simulink model "test_firs"  (Simulink 6.2)
settings: Solver=ode45  StartTime=0.0  StopTime=500  RelTol=1e-3
undefined symbols (not defined in the file or in its folder): now, pfb_coefs
libraries: xbsIndex_r3 x151, pfb_library x1, simulink x1
(part 3 of 3)

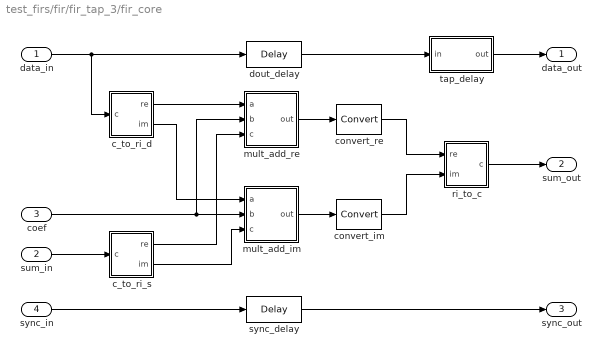
== system test_firs/fir/fir_tap_3/fir_core ==
  data_in : Inport  Port=1  LatchInput=off
  sum_in : Inport  Port=2  LatchInput=off
  coef : Inport  Port=3  LatchInput=off
  sync_in : Inport  Port=4  LatchInput=off
  c_to_ri_d : Subsystem  mask(Complex to Real-Imag){n_bits=8, bin_pt=7}
      mask prompts: n_bits "Bit Width"; bin_pt "Binary Point"
      mask help: Outputs real and imaginary components of a complex input.
      settings: AttributesFormatString=8_7 r/i
      mask Help:
      | <pre>
      | Description::
      | 
      | Outputs real and imaginary components of a complex input.
      | Useful for simplifying interconnects.
      | See also: Real-Imag to Complex (ri_to_c)
      | 
      | Mask Parameters::
      | 
      | Bit Width (n_bits): Specifies the width of the real/imaginary components.
      | Assumed equal for both components.
      | 
      | Binary Point (bin_pt): Specifies the binary point location in the real/imaginary components.
      | Assumed equal for both components.
      | </pre>
  c_to_ri_s : Subsystem  mask(Complex to Real-Imag){n_bits=17, bin_pt=15}
      mask prompts: n_bits "Bit Width"; bin_pt "Binary Point"
      mask help: Outputs real and imaginary components of a complex input.
      settings: AttributesFormatString=17_15 r/i
      mask Help:
      | <pre>
      | Description::
      | 
      | Outputs real and imaginary components of a complex input.
      | Useful for simplifying interconnects.
      | See also: Real-Imag to Complex (ri_to_c)
      | 
      | Mask Parameters::
      | 
      | Bit Width (n_bits): Specifies the width of the real/imaginary components.
      | Assumed equal for both components.
      | 
      | Binary Point (bin_pt): Specifies the binary point location in the real/imaginary components.
      | Assumed equal for both components.
      | </pre>
  convert_im : xbsIndex_r3/Convert  arith_type="Signed  (2's comp)"  n_bits=17  bin_pt=15  quantization=Truncate  overflow=Wrap  latency=0  explicit_period=off  period=1  dbl_ovrd=off  show_param=on  inserted_by_tool=off  pipeline=on
      settings: xl_area=[0, 0, 0, 0, 0, 0, 0]
  convert_re : xbsIndex_r3/Convert  arith_type="Signed  (2's comp)"  n_bits=17  bin_pt=15  quantization=Truncate  overflow=Wrap  latency=0  explicit_period=off  period=1  dbl_ovrd=off  show_param=on  inserted_by_tool=off  pipeline=on
      settings: xl_area=[0, 0, 0, 0, 0, 0, 0]
  dout_delay : xbsIndex_r3/Delay  latency=4  reg_retiming=off  explicit_period=off  period=1  en=off  accept_only_valid=off  init_zero=on  dbl_ovrd=off  show_param=off
      settings: xl_area=[0, 0, 0, 0, 0, 0, 0]
  mult_add_im : Subsystem  mask(Multiply Add Block){mult_latency=3, add_latency=1, add_bypass=off}
      mask prompts: mult_latency "Multiplier Latency"; add_latency "Adder Latency"; add_bypass "Bypass Adder"
      mask help: A full precision multiply-add block. Produces a*b+c at its ab_c output. The add operation can be optionally bypassed.
      settings: AttributesFormatString=|
      | out = a*b+c
      | latency = 4
      mask Help:
      | <pre>
      | Description::
      | 
      | This full precision multiply-add block produces a*b+c at its ab_c output.
      | The add operation can be optionally bypassed.
      | 
      | Latency is one multiplier latency plus one adder latency (if not bypassing adder).
      | 
      | Mask Parameters::
      | 
      | Multiplier Latency (mult_latency): Latency to use for the underlying real multipliers.
      | 
      | Adder Latency (add_latency): Latency to use for the underlying real adders.
      | 
      | Bypass Adder (add_bypass): Check this checkbox to bypass the adder.
      | </pre>
  mult_add_re : Subsystem  mask(Multiply Add Block){mult_latency=3, add_latency=1, add_bypass=off}
      mask prompts: mult_latency "Multiplier Latency"; add_latency "Adder Latency"; add_bypass "Bypass Adder"
      mask help: A full precision multiply-add block. Produces a*b+c at its ab_c output. The add operation can be optionally bypassed.
      settings: AttributesFormatString=|
      | out = a*b+c
      | latency = 4
      mask Help:
      | <pre>
      | Description::
      | 
      | This full precision multiply-add block produces a*b+c at its ab_c output.
      | The add operation can be optionally bypassed.
      | 
      | Latency is one multiplier latency plus one adder latency (if not bypassing adder).
      | 
      | Mask Parameters::
      | 
      | Multiplier Latency (mult_latency): Latency to use for the underlying real multipliers.
      | 
      | Adder Latency (add_latency): Latency to use for the underlying real adders.
      | 
      | Bypass Adder (add_bypass): Check this checkbox to bypass the adder.
      | </pre>
  ri_to_c : Subsystem  mask(Real-Imag to Complex){}
      mask help: Concatenates real and imaginary inputs into a complex output.
      mask init:
      | ri_to_c_init(gcb);
      mask Help:
      | <pre>
      | Description::
      | 
      | Concatenates a real and imaginary input into a complex output.
      | Useful for simplifying interconnects.
      | See also: Complex to Real-Imag (c_to_ri)
      | 
      | Mask Parameters::
      | 
      | (N/A)
      | </pre>
  sync_delay : xbsIndex_r3/Delay  latency=4  reg_retiming=off  explicit_period=off  period=1  en=off  accept_only_valid=off  init_zero=on  dbl_ovrd=off  show_param=off
      settings: xl_area=[0, 0, 0, 0, 0, 0, 0]
  tap_delay : Subsystem  mask(BRAM Delay){delay_depth=64, buffer_latency=}
      mask prompts: delay_depth "Delay Depth"; buffer_latency "Buffer Latency"
      mask help: A delay block that uses BRAM for its storage.
      settings: AttributesFormatString=bram depth = 64
      mask Help:
      | <pre>
      | Description::
      | 
      | A delay block that uses BRAM for its storage.
      | 
      | Mask Parameters::
      | 
      | Delay Depth (delay_depth): The length of the delay.
      | 
      | Buffer Latency (buffer_latency): The latency of the underlying storage.
      | 
      | Buffer Latency defaults to 1 and cannot be changed via the block's dialog box.
      | Future versions may enable the setting of that parameter from the dialog.
      | </pre>
  data_out : Outport
  sum_out : Outport  Port=2
  sync_out : Outport  Port=3
  wires:
  convert_im/1 -> ri_to_c/2(im)
  convert_re/1 -> ri_to_c/1(re)
  tap_delay/1(out) -> data_out/1
  mult_add_im/1(out) -> convert_im/1
  mult_add_re/1(out) -> convert_re/1
  c_to_ri_s/2(im) -> mult_add_im/3(c)
  c_to_ri_s/1(re) -> mult_add_re/3(c)
  sum_in/1 -> c_to_ri_s/1(c)
  coef/1 -> mult_add_re/2(b), mult_add_im/2(b)
  c_to_ri_d/2(im) -> mult_add_im/1(a)
  c_to_ri_d/1(re) -> mult_add_re/1(a)
  data_in/1 -> c_to_ri_d/1(c), dout_delay/1
  dout_delay/1 -> tap_delay/1(in)
  ri_to_c/1(c) -> sum_out/1
  sync_delay/1 -> sync_out/1
  sync_in/1 -> sync_delay/1

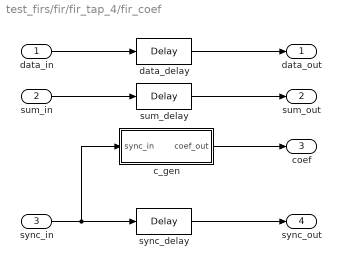
== system test_firs/fir/fir_tap_4/fir_coef ==
  data_in : Inport  Port=1  LatchInput=off
  sum_in : Inport  Port=2  LatchInput=off
  sync_in : Inport  Port=3  LatchInput=off
  c_gen : Subsystem  mask(Coefficient Generator){coefs=[-0.000313693993479576;-0.000949413894136895;-0.00160072502983972;-0.00227308910223182;-0.00297201531120363;-0.00370300584524142;-0.00447149996896613;-0.00528281700660057;-0.0061420985300509;-0.0070542500687595;-0.00802388266542662;-0.00905525460705801;-0.0101522136645361;-0.0113181401759998;-0.0125558913097251;-0.0138677468409146;-0.0152553567738119;-0.0167196911358607;-0.018260992264242;-0.0198787298970449;-0.0215715593716044;-0.0233372832211883;-0.0251728164482839;-0.0270741557382724;-0.0290363528613422;-0.0310534924931389;-0.0331186746659681;-0.035224002042413;-0.0373605721821118;-0.039518474950235;-0.0416867951930131;-0.0438536207815986;-0.0460060561007039;-0.0481302410329562;-0.050211375463868;-0.0522337493058552;-0.0541807780129703;-0.0560350435310833;-0.057778340601254;-0.0593917283071436;-0.0608555867306188;-0.0621496785533557;-0.063253215416367;-0.0641449288240917;-0.064803145355121;-0.0652058659179099;-0.0653308487670656;-0.0651556959741166;-0.0646579430261756;-0.0638151512067052;-0.0626050023947942;-0.0610053959030371;-0.0589945469593747;-0.0565510864251856;-0.0536541613305752;-0.0502835357982813;-0.0464196919199395;-0.0420439301426944;-0.0371384687203353;-0.03168654178132;-0.0256724955662416;-0.0190818823895147;-0.0119015518843096;-0.00411973909604202], n_bits=9, bin_pt=8, log2_cpc=0, use_bram=on}
      mask prompts: coefs "Coefficients"; n_bits "Number of Bits"; bin_pt "Binary Point"; log2_cpc "Log2 Cycles per Coefficient"; use_bram "Use BRAM"
      mask help: A coefficient generator.
      settings: AttributesFormatString=|
      | 64 coefs in bram
      | 9_8 out/1
      mask Help:
      | <pre>
      | Description::
      | 
      | A coefficient generator.
      | 
      | Mask Parameters::
      | 
      | Coefficiants (coefs): The coefficients to output.  These should be specified as doubles.
      | They will be rounded/saturated according to the specified number of bits (n_bits)
      | and binary point (bin_pt).
      | 
      | Number of Coefficient Bits (n_bits): The number of bits used for the fixed point binary
      | representation of the coefficients.
      | 
      | Coefficient Binary Point (bin_pt): The binary point of the fixed point binary representation
      | of the coefficients.
      | 
      | Log2 Cycles per Coefficient (log2_cpc): The log2 value of the number of cycles per coefficient.
      | Must be a non-negative integer (i.e. cycles per coefficient must be a power of 2).
      | 
      | Use BRAM (use_bram): Check this checkbox to store coefficients in BRAM.
      | If unchecked, the coefficients will be sored in distributed memory (i.e. slices).
      | </pre>
  data_delay : xbsIndex_r3/Delay  latency=1  reg_retiming=off  explicit_period=off  period=1  en=off  accept_only_valid=off  init_zero=on  dbl_ovrd=off  show_param=on
      settings: xl_area=[0, 0, 0, 0, 0, 0, 0]
  sum_delay : xbsIndex_r3/Delay  latency=1  reg_retiming=off  explicit_period=off  period=1  en=off  accept_only_valid=off  init_zero=on  dbl_ovrd=off  show_param=on
      settings: xl_area=[0, 0, 0, 0, 0, 0, 0]
  sync_delay : xbsIndex_r3/Delay  latency=1  reg_retiming=off  explicit_period=off  period=1  en=off  accept_only_valid=off  init_zero=on  dbl_ovrd=off  show_param=off
      settings: xl_area=[0, 0, 0, 0, 0, 0, 0]
  data_out : Outport
  sum_out : Outport  Port=2
  coef : Outport  Port=3
  sync_out : Outport  Port=4
  wires:
  c_gen/1(coef_out) -> coef/1
  sum_delay/1 -> sum_out/1
  sum_in/1 -> sum_delay/1
  sync_in/1 -> c_gen/1(sync_in), sync_delay/1
  sync_delay/1 -> sync_out/1
  data_delay/1 -> data_out/1
  data_in/1 -> data_delay/1

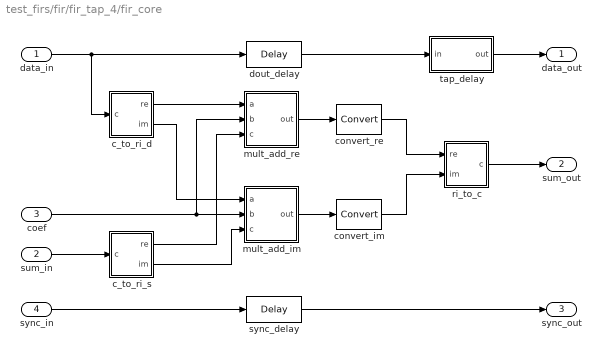
== system test_firs/fir/fir_tap_4/fir_core ==
  data_in : Inport  Port=1  LatchInput=off
  sum_in : Inport  Port=2  LatchInput=off
  coef : Inport  Port=3  LatchInput=off
  sync_in : Inport  Port=4  LatchInput=off
  c_to_ri_d : Subsystem  mask(Complex to Real-Imag){n_bits=8, bin_pt=7}
      mask prompts: n_bits "Bit Width"; bin_pt "Binary Point"
      mask help: Outputs real and imaginary components of a complex input.
      settings: AttributesFormatString=8_7 r/i
      mask Help:
      | <pre>
      | Description::
      | 
      | Outputs real and imaginary components of a complex input.
      | Useful for simplifying interconnects.
      | See also: Real-Imag to Complex (ri_to_c)
      | 
      | Mask Parameters::
      | 
      | Bit Width (n_bits): Specifies the width of the real/imaginary components.
      | Assumed equal for both components.
      | 
      | Binary Point (bin_pt): Specifies the binary point location in the real/imaginary components.
      | Assumed equal for both components.
      | </pre>
  c_to_ri_s : Subsystem  mask(Complex to Real-Imag){n_bits=17, bin_pt=15}
      mask prompts: n_bits "Bit Width"; bin_pt "Binary Point"
      mask help: Outputs real and imaginary components of a complex input.
      settings: AttributesFormatString=17_15 r/i
      mask Help:
      | <pre>
      | Description::
      | 
      | Outputs real and imaginary components of a complex input.
      | Useful for simplifying interconnects.
      | See also: Real-Imag to Complex (ri_to_c)
      | 
      | Mask Parameters::
      | 
      | Bit Width (n_bits): Specifies the width of the real/imaginary components.
      | Assumed equal for both components.
      | 
      | Binary Point (bin_pt): Specifies the binary point location in the real/imaginary components.
      | Assumed equal for both components.
      | </pre>
  convert_im : xbsIndex_r3/Convert  arith_type="Signed  (2's comp)"  n_bits=17  bin_pt=15  quantization=Truncate  overflow=Wrap  latency=0  explicit_period=off  period=1  dbl_ovrd=off  show_param=on  inserted_by_tool=off  pipeline=on
      settings: xl_area=[0, 0, 0, 0, 0, 0, 0]
  convert_re : xbsIndex_r3/Convert  arith_type="Signed  (2's comp)"  n_bits=17  bin_pt=15  quantization=Truncate  overflow=Wrap  latency=0  explicit_period=off  period=1  dbl_ovrd=off  show_param=on  inserted_by_tool=off  pipeline=on
      settings: xl_area=[0, 0, 0, 0, 0, 0, 0]
  dout_delay : xbsIndex_r3/Delay  latency=4  reg_retiming=off  explicit_period=off  period=1  en=off  accept_only_valid=off  init_zero=on  dbl_ovrd=off  show_param=off
      settings: xl_area=[0, 0, 0, 0, 0, 0, 0]
  mult_add_im : Subsystem  mask(Multiply Add Block){mult_latency=3, add_latency=1, add_bypass=off}
      mask prompts: mult_latency "Multiplier Latency"; add_latency "Adder Latency"; add_bypass "Bypass Adder"
      mask help: A full precision multiply-add block. Produces a*b+c at its ab_c output. The add operation can be optionally bypassed.
      settings: AttributesFormatString=|
      | out = a*b+c
      | latency = 4
      mask Help:
      | <pre>
      | Description::
      | 
      | This full precision multiply-add block produces a*b+c at its ab_c output.
      | The add operation can be optionally bypassed.
      | 
      | Latency is one multiplier latency plus one adder latency (if not bypassing adder).
      | 
      | Mask Parameters::
      | 
      | Multiplier Latency (mult_latency): Latency to use for the underlying real multipliers.
      | 
      | Adder Latency (add_latency): Latency to use for the underlying real adders.
      | 
      | Bypass Adder (add_bypass): Check this checkbox to bypass the adder.
      | </pre>
  mult_add_re : Subsystem  mask(Multiply Add Block){mult_latency=3, add_latency=1, add_bypass=off}
      mask prompts: mult_latency "Multiplier Latency"; add_latency "Adder Latency"; add_bypass "Bypass Adder"
      mask help: A full precision multiply-add block. Produces a*b+c at its ab_c output. The add operation can be optionally bypassed.
      settings: AttributesFormatString=|
      | out = a*b+c
      | latency = 4
      mask Help:
      | <pre>
      | Description::
      | 
      | This full precision multiply-add block produces a*b+c at its ab_c output.
      | The add operation can be optionally bypassed.
      | 
      | Latency is one multiplier latency plus one adder latency (if not bypassing adder).
      | 
      | Mask Parameters::
      | 
      | Multiplier Latency (mult_latency): Latency to use for the underlying real multipliers.
      | 
      | Adder Latency (add_latency): Latency to use for the underlying real adders.
      | 
      | Bypass Adder (add_bypass): Check this checkbox to bypass the adder.
      | </pre>
  ri_to_c : Subsystem  mask(Real-Imag to Complex){}
      mask help: Concatenates real and imaginary inputs into a complex output.
      mask init:
      | ri_to_c_init(gcb);
      mask Help:
      | <pre>
      | Description::
      | 
      | Concatenates a real and imaginary input into a complex output.
      | Useful for simplifying interconnects.
      | See also: Complex to Real-Imag (c_to_ri)
      | 
      | Mask Parameters::
      | 
      | (N/A)
      | </pre>
  sync_delay : xbsIndex_r3/Delay  latency=4  reg_retiming=off  explicit_period=off  period=1  en=off  accept_only_valid=off  init_zero=on  dbl_ovrd=off  show_param=off
      settings: xl_area=[0, 0, 0, 0, 0, 0, 0]
  tap_delay : Subsystem  mask(SLR16 Delay){delay_depth=0}
      mask prompts: delay_depth "Delay Depth"
      mask help: A delay block that uses SLR16 elements for its storage.
      settings: AttributesFormatString=slr depth = 0
      mask Help:
      | <pre>
      | Description::
      | 
      | A delay block that uses SLR16 elements for its storage.
      | 
      | Mask Parameters::
      | 
      | Delay Depth (delay_depth): The length of the delay.
      | </pre>
  data_out : Outport
  sum_out : Outport  Port=2
  sync_out : Outport  Port=3
  wires:
  convert_im/1 -> ri_to_c/2(im)
  convert_re/1 -> ri_to_c/1(re)
  tap_delay/1(out) -> data_out/1
  mult_add_im/1(out) -> convert_im/1
  mult_add_re/1(out) -> convert_re/1
  c_to_ri_s/2(im) -> mult_add_im/3(c)
  c_to_ri_s/1(re) -> mult_add_re/3(c)
  sum_in/1 -> c_to_ri_s/1(c)
  coef/1 -> mult_add_re/2(b), mult_add_im/2(b)
  c_to_ri_d/2(im) -> mult_add_im/1(a)
  c_to_ri_d/1(re) -> mult_add_re/1(a)
  data_in/1 -> c_to_ri_d/1(c), dout_delay/1
  dout_delay/1 -> tap_delay/1(in)
  ri_to_c/1(c) -> sum_out/1
  sync_delay/1 -> sync_out/1
  sync_in/1 -> sync_delay/1

== system test_firs/fir/fir_tap_1/fir_coef/c_gen ==
  sync_in : Inport  Port=1  LatchInput=off
  Counter : xbsIndex_r3/Counter  cnt_type=Count Limited  n_bits=6  bin_pt=0  arith_type=Unsigned  start_count=0  cnt_to=63  cnt_by_val=1  operation=Up  explicit_period=off  period=1  load_pin=off  rst=on  en=off  dbl_ovrd=off  show_param=on  use_rpm=on  gen_core=off
      settings: xl_area=[0, 0, 0, 0, 0, 0, 0]
  addr_sel : xbsIndex_r3/Slice  mode=Upper Bit Location + Width  nbits=6  bit1=0  base1=MSB of Input  bit0=-1  base0=MSB of Input  boolean_output=off  explicit_period=off  period=1  dbl_ovrd=off
  mem : xbsIndex_r3/ROM  depth=64  initVector=[-0.00390625;-0.01171875;-0.01953125;-0.02734375;-0.03125;-0.0390625;-0.04296875;-0.046875;-0.05078125;-0.0546875;-0.0546875;-0.05859375;-0.0625;-0.0625;-0.0625;-0.06640625;-0.06640625;-0.06640625;-0.06640625;-0.06640625;-0.0625;-0.0625;-0.0625;-0.0625;-0.05859375;-0.05859375;-0.0546875;-0.0546875;-0.05078125;-0.05078125;-0.046875;-0.046875;-0.04296875;-0.04296875;-0.0390625;-0.0390625;-0.03515625;-0.03125;-0.03125;-0.02734375;-0.02734375;-0.0234375;-0.0234375;-0.0234375;-0.01953125;-0.01953125;-0.015625;-0.015625;-0.015625;-0.01171875;-0.01171875;-0.01171875;-0.0078125;-0.0078125;-0.0078125;-0.0078125;-0.00390625;-0.00390625;-0.00390625;-0.00390625;-0.00390625;0;0;0]  arith_type="Signed  (2's comp)"  n_bits=9  bin_pt=8  latency=1  init_zero=on  explicit_period=off  period=1  rst=off  init_reg=0  en=off  dbl_ovrd=off  show_param=on  distributed_mem=off  use_rpm=on  gen_core=off
      settings: AttributesFormatString=depth = %<depth>\ndist_mem = %<distributed_mem>  xl_area=[0, 0, 0, 0, 0, 0, 0]
  coef_out : Outport
  wires:
  sync_in/1 -> Counter/1
  Counter/1 -> addr_sel/1
  addr_sel/1 -> mem/1
  mem/1 -> coef_out/1

== system test_firs/fir/fir_tap_1/fir_core/c_to_ri_d ==
  c : Inport  Port=1  LatchInput=off
  force_im : xbsIndex_r3/Reinterpret  force_arith_type=on  arith_type="Signed  (2's comp)"  force_bin_pt=on  bin_pt=7  force_valid=on
  force_re : xbsIndex_r3/Reinterpret  force_arith_type=on  arith_type="Signed  (2's comp)"  force_bin_pt=on  bin_pt=7  force_valid=on
  slice_im : xbsIndex_r3/Slice  mode=Lower Bit Location + Width  nbits=8  bit1=0  base1=MSB of Input  bit0=0  base0=LSB of Input  boolean_output=off  explicit_period=off  period=1  dbl_ovrd=off
  slice_re : xbsIndex_r3/Slice  mode=Upper Bit Location + Width  nbits=8  bit1=0  base1=MSB of Input  bit0=0  base0=LSB of Input  boolean_output=off  explicit_period=off  period=1  dbl_ovrd=off
  re : Outport
  im : Outport  Port=2
  wires:
  slice_re/1 -> force_re/1
  slice_im/1 -> force_im/1
  force_re/1 -> re/1
  force_im/1 -> im/1
  c/1 -> slice_re/1, slice_im/1

== system test_firs/fir/fir_tap_1/fir_core/c_to_ri_s ==
  c : Inport  Port=1  LatchInput=off
  force_im : xbsIndex_r3/Reinterpret  force_arith_type=on  arith_type="Signed  (2's comp)"  force_bin_pt=on  bin_pt=15  force_valid=on
  force_re : xbsIndex_r3/Reinterpret  force_arith_type=on  arith_type="Signed  (2's comp)"  force_bin_pt=on  bin_pt=15  force_valid=on
  slice_im : xbsIndex_r3/Slice  mode=Lower Bit Location + Width  nbits=17  bit1=0  base1=MSB of Input  bit0=0  base0=LSB of Input  boolean_output=off  explicit_period=off  period=1  dbl_ovrd=off
  slice_re : xbsIndex_r3/Slice  mode=Upper Bit Location + Width  nbits=17  bit1=0  base1=MSB of Input  bit0=0  base0=LSB of Input  boolean_output=off  explicit_period=off  period=1  dbl_ovrd=off
  re : Outport
  im : Outport  Port=2
  wires:
  slice_re/1 -> force_re/1
  slice_im/1 -> force_im/1
  force_re/1 -> re/1
  force_im/1 -> im/1
  c/1 -> slice_re/1, slice_im/1

== system test_firs/fir/fir_tap_1/fir_core/mult_add_im ==
  a : Inport  Port=1  LatchInput=off
  b : Inport  Port=2  LatchInput=off
  c : Inport  Port=3  LatchInput=off
  Terminator : Terminator
  add : xbsIndex_r3/AddSub  mode=Addition  precision=User Defined  arith_type="Signed  (2's comp)"  n_bits=9  bin_pt=7  quantization=Truncate  overflow=Wrap  latency=1  explicit_period=off  period=1  use_carryin=off  use_carryout=off  en=off  dbl_ovrd=off  show_param=on  use_core=on  pipeline=on  use_rpm=on  gen_core=off
      settings: xl_area=[0, 0, 0, 0, 0, 0, 0]
  delay : xbsIndex_r3/Delay  latency=3  reg_retiming=off  explicit_period=off  period=1  en=off  accept_only_valid=off  init_zero=on  dbl_ovrd=off  show_param=off
      settings: xl_area=[0, 0, 0, 0, 0, 0, 0]
  mult : xbsIndex_r3/Mult  precision=Full  arith_type="Signed  (2's comp)"  n_bits=8  bin_pt=2  quantization=Truncate  overflow=Wrap  latency=3  explicit_period=off  period=1  en=off  dbl_ovrd=off  show_param=on  mult_type=Parallel  oversample=2  use_embedded=on  pipeline=on  use_rpm=on  placement_style=Rectangular Shape  gen_core=off
      settings: xl_area=[0, 0, 0, 0, 0, 0, 0]
  out : Outport
  wires:
  mult/1 -> add/1, out/1
  delay/1 -> add/2
  a/1 -> mult/1
  b/1 -> mult/2
  c/1 -> delay/1
  add/1 -> Terminator/1

== system test_firs/fir/fir_tap_1/fir_core/mult_add_re ==
  a : Inport  Port=1  LatchInput=off
  b : Inport  Port=2  LatchInput=off
  c : Inport  Port=3  LatchInput=off
  Terminator : Terminator
  add : xbsIndex_r3/AddSub  mode=Addition  precision=User Defined  arith_type="Signed  (2's comp)"  n_bits=9  bin_pt=7  quantization=Truncate  overflow=Wrap  latency=1  explicit_period=off  period=1  use_carryin=off  use_carryout=off  en=off  dbl_ovrd=off  show_param=on  use_core=on  pipeline=on  use_rpm=on  gen_core=off
      settings: xl_area=[0, 0, 0, 0, 0, 0, 0]
  delay : xbsIndex_r3/Delay  latency=3  reg_retiming=off  explicit_period=off  period=1  en=off  accept_only_valid=off  init_zero=on  dbl_ovrd=off  show_param=off
      settings: xl_area=[0, 0, 0, 0, 0, 0, 0]
  mult : xbsIndex_r3/Mult  precision=Full  arith_type="Signed  (2's comp)"  n_bits=8  bin_pt=2  quantization=Truncate  overflow=Wrap  latency=3  explicit_period=off  period=1  en=off  dbl_ovrd=off  show_param=on  mult_type=Parallel  oversample=2  use_embedded=on  pipeline=on  use_rpm=on  placement_style=Rectangular Shape  gen_core=off
      settings: xl_area=[0, 0, 0, 0, 0, 0, 0]
  out : Outport
  wires:
  mult/1 -> add/1, out/1
  delay/1 -> add/2
  a/1 -> mult/1
  b/1 -> mult/2
  c/1 -> delay/1
  add/1 -> Terminator/1

== system test_firs/fir/fir_tap_1/fir_core/ri_to_c ==
  re : Inport  Port=1  LatchInput=off
  im : Inport  Port=2  LatchInput=off
  concat : xbsIndex_r3/Concat  num_inputs=2  explicit_period=off  period=1  dbl_ovrd=off
  force_im : xbsIndex_r3/Reinterpret  force_arith_type=on  arith_type=Unsigned  force_bin_pt=on  bin_pt=0  force_valid=on
  force_re : xbsIndex_r3/Reinterpret  force_arith_type=on  arith_type=Unsigned  force_bin_pt=on  bin_pt=0  force_valid=on
  c : Outport
  wires:
  im/1 -> force_im/1
  concat/1 -> c/1
  re/1 -> force_re/1
  force_im/1 -> concat/2
  force_re/1 -> concat/1

== system test_firs/fir/fir_tap_1/fir_core/tap_delay ==
  in : Inport  Port=1  LatchInput=off
  Constant : xbsIndex_r3/Constant  const=1  equ=P=C  arith_type=Boolean  n_bits=1  bin_pt=0  opselect=C  inp2=PCIN>>17  opr=+  inp1=P  carry=CIN  iostate=0  explicit_period=on  period=1  dbl_ovrd=off
  Counter : xbsIndex_r3/Counter  cnt_type=Count Limited  n_bits=6  bin_pt=0  arith_type=Unsigned  start_count=0  cnt_to=62  cnt_by_val=1  operation=Up  explicit_period=off  period=1  load_pin=off  rst=off  en=off  dbl_ovrd=off  show_param=off  use_rpm=on  gen_core=off
      settings: xl_area=[0, 0, 0, 0, 0, 0, 0]
  bram : xbsIndex_r3/Single Port RAM  depth=64  initVector=0  write_mode=Read Before Write  latency=1  init_zero=on  explicit_period=off  period=1  rst=off  init_reg=0  en=off  dbl_ovrd=off  show_param=off  distributed_mem=off  use_rpm=off  gen_core=off
      settings: xl_area=[0, 0, 0, 0, 0, 0, 0]
  out : Outport
  wires:
  Constant/1 -> bram/3
  in/1 -> bram/2
  bram/1 -> out/1
  Counter/1 -> bram/1

== system test_firs/fir/fir_tap_2/fir_coef/c_gen ==
  sync_in : Inport  Port=1  LatchInput=off
  Counter : xbsIndex_r3/Counter  cnt_type=Count Limited  n_bits=6  bin_pt=0  arith_type=Unsigned  start_count=0  cnt_to=63  cnt_by_val=1  operation=Up  explicit_period=off  period=1  load_pin=off  rst=on  en=off  dbl_ovrd=off  show_param=on  use_rpm=on  gen_core=off
      settings: xl_area=[0, 0, 0, 0, 0, 0, 0]
  addr_sel : xbsIndex_r3/Slice  mode=Upper Bit Location + Width  nbits=6  bit1=0  base1=MSB of Input  bit0=-1  base0=MSB of Input  boolean_output=off  explicit_period=off  period=1  dbl_ovrd=off
  mem : xbsIndex_r3/ROM  depth=64  initVector=[0.99609375;0.99609375;0.99609375;0.9921875;0.98828125;0.984375;0.9765625;0.96875;0.9609375;0.953125;0.94140625;0.9296875;0.91796875;0.90625;0.890625;0.875;0.859375;0.84375;0.828125;0.80859375;0.79296875;0.7734375;0.75390625;0.734375;0.7109375;0.69140625;0.671875;0.6484375;0.62890625;0.60546875;0.58203125;0.5625;0.5390625;0.515625;0.49609375;0.47265625;0.44921875;0.4296875;0.40625;0.3828125;0.36328125;0.34375;0.3203125;0.30078125;0.28125;0.26171875;0.2421875;0.22265625;0.20703125;0.1875;0.171875;0.15234375;0.13671875;0.12109375;0.109375;0.09375;0.08203125;0.06640625;0.0546875;0.04296875;0.03515625;0.0234375;0.01171875;0.00390625]  arith_type="Signed  (2's comp)"  n_bits=9  bin_pt=8  latency=1  init_zero=on  explicit_period=off  period=1  rst=off  init_reg=0  en=off  dbl_ovrd=off  show_param=on  distributed_mem=off  use_rpm=on  gen_core=off
      settings: AttributesFormatString=depth = %<depth>\ndist_mem = %<distributed_mem>  xl_area=[0, 0, 0, 0, 0, 0, 0]
  coef_out : Outport
  wires:
  sync_in/1 -> Counter/1
  Counter/1 -> addr_sel/1
  addr_sel/1 -> mem/1
  mem/1 -> coef_out/1

== system test_firs/fir/fir_tap_2/fir_core/c_to_ri_d ==
  c : Inport  Port=1  LatchInput=off
  force_im : xbsIndex_r3/Reinterpret  force_arith_type=on  arith_type="Signed  (2's comp)"  force_bin_pt=on  bin_pt=7  force_valid=on
  force_re : xbsIndex_r3/Reinterpret  force_arith_type=on  arith_type="Signed  (2's comp)"  force_bin_pt=on  bin_pt=7  force_valid=on
  slice_im : xbsIndex_r3/Slice  mode=Lower Bit Location + Width  nbits=8  bit1=0  base1=MSB of Input  bit0=0  base0=LSB of Input  boolean_output=off  explicit_period=off  period=1  dbl_ovrd=off
  slice_re : xbsIndex_r3/Slice  mode=Upper Bit Location + Width  nbits=8  bit1=0  base1=MSB of Input  bit0=0  base0=LSB of Input  boolean_output=off  explicit_period=off  period=1  dbl_ovrd=off
  re : Outport
  im : Outport  Port=2
  wires:
  slice_re/1 -> force_re/1
  slice_im/1 -> force_im/1
  force_re/1 -> re/1
  force_im/1 -> im/1
  c/1 -> slice_re/1, slice_im/1

== system test_firs/fir/fir_tap_2/fir_core/c_to_ri_s ==
  c : Inport  Port=1  LatchInput=off
  force_im : xbsIndex_r3/Reinterpret  force_arith_type=on  arith_type="Signed  (2's comp)"  force_bin_pt=on  bin_pt=15  force_valid=on
  force_re : xbsIndex_r3/Reinterpret  force_arith_type=on  arith_type="Signed  (2's comp)"  force_bin_pt=on  bin_pt=15  force_valid=on
  slice_im : xbsIndex_r3/Slice  mode=Lower Bit Location + Width  nbits=17  bit1=0  base1=MSB of Input  bit0=0  base0=LSB of Input  boolean_output=off  explicit_period=off  period=1  dbl_ovrd=off
  slice_re : xbsIndex_r3/Slice  mode=Upper Bit Location + Width  nbits=17  bit1=0  base1=MSB of Input  bit0=0  base0=LSB of Input  boolean_output=off  explicit_period=off  period=1  dbl_ovrd=off
  re : Outport
  im : Outport  Port=2
  wires:
  slice_re/1 -> force_re/1
  slice_im/1 -> force_im/1
  force_re/1 -> re/1
  force_im/1 -> im/1
  c/1 -> slice_re/1, slice_im/1

== system test_firs/fir/fir_tap_2/fir_core/mult_add_im ==
  a : Inport  Port=1  LatchInput=off
  b : Inport  Port=2  LatchInput=off
  c : Inport  Port=3  LatchInput=off
  add : xbsIndex_r3/AddSub  mode=Addition  precision=User Defined  arith_type="Signed  (2's comp)"  n_bits=9  bin_pt=7  quantization=Truncate  overflow=Wrap  latency=1  explicit_period=off  period=1  use_carryin=off  use_carryout=off  en=off  dbl_ovrd=off  show_param=on  use_core=on  pipeline=on  use_rpm=on  gen_core=off
      settings: xl_area=[0, 0, 0, 0, 0, 0, 0]
  delay : xbsIndex_r3/Delay  latency=3  reg_retiming=off  explicit_period=off  period=1  en=off  accept_only_valid=off  init_zero=on  dbl_ovrd=off  show_param=off
      settings: xl_area=[0, 0, 0, 0, 0, 0, 0]
  mult : xbsIndex_r3/Mult  precision=Full  arith_type="Signed  (2's comp)"  n_bits=8  bin_pt=2  quantization=Truncate  overflow=Wrap  latency=3  explicit_period=off  period=1  en=off  dbl_ovrd=off  show_param=on  mult_type=Parallel  oversample=2  use_embedded=on  pipeline=on  use_rpm=on  placement_style=Rectangular Shape  gen_core=off
      settings: xl_area=[0, 0, 0, 0, 0, 0, 0]
  out : Outport
  wires:
  add/1 -> out/1
  mult/1 -> add/1
  delay/1 -> add/2
  a/1 -> mult/1
  b/1 -> mult/2
  c/1 -> delay/1

== system test_firs/fir/fir_tap_2/fir_core/mult_add_re ==
  a : Inport  Port=1  LatchInput=off
  b : Inport  Port=2  LatchInput=off
  c : Inport  Port=3  LatchInput=off
  add : xbsIndex_r3/AddSub  mode=Addition  precision=User Defined  arith_type="Signed  (2's comp)"  n_bits=9  bin_pt=7  quantization=Truncate  overflow=Wrap  latency=1  explicit_period=off  period=1  use_carryin=off  use_carryout=off  en=off  dbl_ovrd=off  show_param=on  use_core=on  pipeline=on  use_rpm=on  gen_core=off
      settings: xl_area=[0, 0, 0, 0, 0, 0, 0]
  delay : xbsIndex_r3/Delay  latency=3  reg_retiming=off  explicit_period=off  period=1  en=off  accept_only_valid=off  init_zero=on  dbl_ovrd=off  show_param=off
      settings: xl_area=[0, 0, 0, 0, 0, 0, 0]
  mult : xbsIndex_r3/Mult  precision=Full  arith_type="Signed  (2's comp)"  n_bits=8  bin_pt=2  quantization=Truncate  overflow=Wrap  latency=3  explicit_period=off  period=1  en=off  dbl_ovrd=off  show_param=on  mult_type=Parallel  oversample=2  use_embedded=on  pipeline=on  use_rpm=on  placement_style=Rectangular Shape  gen_core=off
      settings: xl_area=[0, 0, 0, 0, 0, 0, 0]
  out : Outport
  wires:
  add/1 -> out/1
  mult/1 -> add/1
  delay/1 -> add/2
  a/1 -> mult/1
  b/1 -> mult/2
  c/1 -> delay/1

== system test_firs/fir/fir_tap_2/fir_core/ri_to_c ==
  re : Inport  Port=1  LatchInput=off
  im : Inport  Port=2  LatchInput=off
  concat : xbsIndex_r3/Concat  num_inputs=2  explicit_period=off  period=1  dbl_ovrd=off
  force_im : xbsIndex_r3/Reinterpret  force_arith_type=on  arith_type=Unsigned  force_bin_pt=on  bin_pt=0  force_valid=on
  force_re : xbsIndex_r3/Reinterpret  force_arith_type=on  arith_type=Unsigned  force_bin_pt=on  bin_pt=0  force_valid=on
  c : Outport
  wires:
  im/1 -> force_im/1
  concat/1 -> c/1
  re/1 -> force_re/1
  force_im/1 -> concat/2
  force_re/1 -> concat/1

== system test_firs/fir/fir_tap_2/fir_core/tap_delay ==
  in : Inport  Port=1  LatchInput=off
  Constant : xbsIndex_r3/Constant  const=1  equ=P=C  arith_type=Boolean  n_bits=1  bin_pt=0  opselect=C  inp2=PCIN>>17  opr=+  inp1=P  carry=CIN  iostate=0  explicit_period=on  period=1  dbl_ovrd=off
  Counter : xbsIndex_r3/Counter  cnt_type=Count Limited  n_bits=6  bin_pt=0  arith_type=Unsigned  start_count=0  cnt_to=62  cnt_by_val=1  operation=Up  explicit_period=off  period=1  load_pin=off  rst=off  en=off  dbl_ovrd=off  show_param=off  use_rpm=on  gen_core=off
      settings: xl_area=[0, 0, 0, 0, 0, 0, 0]
  bram : xbsIndex_r3/Single Port RAM  depth=64  initVector=0  write_mode=Read Before Write  latency=1  init_zero=on  explicit_period=off  period=1  rst=off  init_reg=0  en=off  dbl_ovrd=off  show_param=off  distributed_mem=off  use_rpm=off  gen_core=off
      settings: xl_area=[0, 0, 0, 0, 0, 0, 0]
  out : Outport
  wires:
  Constant/1 -> bram/3
  in/1 -> bram/2
  bram/1 -> out/1
  Counter/1 -> bram/1

== system test_firs/fir/fir_tap_3/fir_coef/c_gen ==
  sync_in : Inport  Port=1  LatchInput=off
  Counter : xbsIndex_r3/Counter  cnt_type=Count Limited  n_bits=6  bin_pt=0  arith_type=Unsigned  start_count=0  cnt_to=63  cnt_by_val=1  operation=Up  explicit_period=off  period=1  load_pin=off  rst=on  en=off  dbl_ovrd=off  show_param=on  use_rpm=on  gen_core=off
      settings: xl_area=[0, 0, 0, 0, 0, 0, 0]
  addr_sel : xbsIndex_r3/Slice  mode=Upper Bit Location + Width  nbits=6  bit1=0  base1=MSB of Input  bit0=-1  base0=MSB of Input  boolean_output=off  explicit_period=off  period=1  dbl_ovrd=off
  mem : xbsIndex_r3/ROM  depth=64  initVector=[0.00390625;0.01171875;0.0234375;0.03515625;0.04296875;0.0546875;0.06640625;0.08203125;0.09375;0.109375;0.12109375;0.13671875;0.15234375;0.171875;0.1875;0.20703125;0.22265625;0.2421875;0.26171875;0.28125;0.30078125;0.3203125;0.34375;0.36328125;0.3828125;0.40625;0.4296875;0.44921875;0.47265625;0.49609375;0.515625;0.5390625;0.5625;0.58203125;0.60546875;0.62890625;0.6484375;0.671875;0.69140625;0.7109375;0.734375;0.75390625;0.7734375;0.79296875;0.80859375;0.828125;0.84375;0.859375;0.875;0.890625;0.90625;0.91796875;0.9296875;0.94140625;0.953125;0.9609375;0.96875;0.9765625;0.984375;0.98828125;0.9921875;0.99609375;0.99609375;0.99609375]  arith_type="Signed  (2's comp)"  n_bits=9  bin_pt=8  latency=1  init_zero=on  explicit_period=off  period=1  rst=off  init_reg=0  en=off  dbl_ovrd=off  show_param=on  distributed_mem=off  use_rpm=on  gen_core=off
      settings: AttributesFormatString=depth = %<depth>\ndist_mem = %<distributed_mem>  xl_area=[0, 0, 0, 0, 0, 0, 0]
  coef_out : Outport
  wires:
  sync_in/1 -> Counter/1
  Counter/1 -> addr_sel/1
  addr_sel/1 -> mem/1
  mem/1 -> coef_out/1

== system test_firs/fir/fir_tap_3/fir_core/c_to_ri_d ==
  c : Inport  Port=1  LatchInput=off
  force_im : xbsIndex_r3/Reinterpret  force_arith_type=on  arith_type="Signed  (2's comp)"  force_bin_pt=on  bin_pt=7  force_valid=on
  force_re : xbsIndex_r3/Reinterpret  force_arith_type=on  arith_type="Signed  (2's comp)"  force_bin_pt=on  bin_pt=7  force_valid=on
  slice_im : xbsIndex_r3/Slice  mode=Lower Bit Location + Width  nbits=8  bit1=0  base1=MSB of Input  bit0=0  base0=LSB of Input  boolean_output=off  explicit_period=off  period=1  dbl_ovrd=off
  slice_re : xbsIndex_r3/Slice  mode=Upper Bit Location + Width  nbits=8  bit1=0  base1=MSB of Input  bit0=0  base0=LSB of Input  boolean_output=off  explicit_period=off  period=1  dbl_ovrd=off
  re : Outport
  im : Outport  Port=2
  wires:
  slice_re/1 -> force_re/1
  slice_im/1 -> force_im/1
  force_re/1 -> re/1
  force_im/1 -> im/1
  c/1 -> slice_re/1, slice_im/1

== system test_firs/fir/fir_tap_3/fir_core/c_to_ri_s ==
  c : Inport  Port=1  LatchInput=off
  force_im : xbsIndex_r3/Reinterpret  force_arith_type=on  arith_type="Signed  (2's comp)"  force_bin_pt=on  bin_pt=15  force_valid=on
  force_re : xbsIndex_r3/Reinterpret  force_arith_type=on  arith_type="Signed  (2's comp)"  force_bin_pt=on  bin_pt=15  force_valid=on
  slice_im : xbsIndex_r3/Slice  mode=Lower Bit Location + Width  nbits=17  bit1=0  base1=MSB of Input  bit0=0  base0=LSB of Input  boolean_output=off  explicit_period=off  period=1  dbl_ovrd=off
  slice_re : xbsIndex_r3/Slice  mode=Upper Bit Location + Width  nbits=17  bit1=0  base1=MSB of Input  bit0=0  base0=LSB of Input  boolean_output=off  explicit_period=off  period=1  dbl_ovrd=off
  re : Outport
  im : Outport  Port=2
  wires:
  slice_re/1 -> force_re/1
  slice_im/1 -> force_im/1
  force_re/1 -> re/1
  force_im/1 -> im/1
  c/1 -> slice_re/1, slice_im/1

== system test_firs/fir/fir_tap_3/fir_core/mult_add_im ==
  a : Inport  Port=1  LatchInput=off
  b : Inport  Port=2  LatchInput=off
  c : Inport  Port=3  LatchInput=off
  add : xbsIndex_r3/AddSub  mode=Addition  precision=User Defined  arith_type="Signed  (2's comp)"  n_bits=9  bin_pt=7  quantization=Truncate  overflow=Wrap  latency=1  explicit_period=off  period=1  use_carryin=off  use_carryout=off  en=off  dbl_ovrd=off  show_param=on  use_core=on  pipeline=on  use_rpm=on  gen_core=off
      settings: xl_area=[0, 0, 0, 0, 0, 0, 0]
  delay : xbsIndex_r3/Delay  latency=3  reg_retiming=off  explicit_period=off  period=1  en=off  accept_only_valid=off  init_zero=on  dbl_ovrd=off  show_param=off
      settings: xl_area=[0, 0, 0, 0, 0, 0, 0]
  mult : xbsIndex_r3/Mult  precision=Full  arith_type="Signed  (2's comp)"  n_bits=8  bin_pt=2  quantization=Truncate  overflow=Wrap  latency=3  explicit_period=off  period=1  en=off  dbl_ovrd=off  show_param=on  mult_type=Parallel  oversample=2  use_embedded=on  pipeline=on  use_rpm=on  placement_style=Rectangular Shape  gen_core=off
      settings: xl_area=[0, 0, 0, 0, 0, 0, 0]
  out : Outport
  wires:
  add/1 -> out/1
  mult/1 -> add/1
  delay/1 -> add/2
  a/1 -> mult/1
  b/1 -> mult/2
  c/1 -> delay/1

== system test_firs/fir/fir_tap_3/fir_core/mult_add_re ==
  a : Inport  Port=1  LatchInput=off
  b : Inport  Port=2  LatchInput=off
  c : Inport  Port=3  LatchInput=off
  add : xbsIndex_r3/AddSub  mode=Addition  precision=User Defined  arith_type="Signed  (2's comp)"  n_bits=9  bin_pt=7  quantization=Truncate  overflow=Wrap  latency=1  explicit_period=off  period=1  use_carryin=off  use_carryout=off  en=off  dbl_ovrd=off  show_param=on  use_core=on  pipeline=on  use_rpm=on  gen_core=off
      settings: xl_area=[0, 0, 0, 0, 0, 0, 0]
  delay : xbsIndex_r3/Delay  latency=3  reg_retiming=off  explicit_period=off  period=1  en=off  accept_only_valid=off  init_zero=on  dbl_ovrd=off  show_param=off
      settings: xl_area=[0, 0, 0, 0, 0, 0, 0]
  mult : xbsIndex_r3/Mult  precision=Full  arith_type="Signed  (2's comp)"  n_bits=8  bin_pt=2  quantization=Truncate  overflow=Wrap  latency=3  explicit_period=off  period=1  en=off  dbl_ovrd=off  show_param=on  mult_type=Parallel  oversample=2  use_embedded=on  pipeline=on  use_rpm=on  placement_style=Rectangular Shape  gen_core=off
      settings: xl_area=[0, 0, 0, 0, 0, 0, 0]
  out : Outport
  wires:
  add/1 -> out/1
  mult/1 -> add/1
  delay/1 -> add/2
  a/1 -> mult/1
  b/1 -> mult/2
  c/1 -> delay/1

== system test_firs/fir/fir_tap_3/fir_core/ri_to_c ==
  re : Inport  Port=1  LatchInput=off
  im : Inport  Port=2  LatchInput=off
  concat : xbsIndex_r3/Concat  num_inputs=2  explicit_period=off  period=1  dbl_ovrd=off
  force_im : xbsIndex_r3/Reinterpret  force_arith_type=on  arith_type=Unsigned  force_bin_pt=on  bin_pt=0  force_valid=on
  force_re : xbsIndex_r3/Reinterpret  force_arith_type=on  arith_type=Unsigned  force_bin_pt=on  bin_pt=0  force_valid=on
  c : Outport
  wires:
  im/1 -> force_im/1
  concat/1 -> c/1
  re/1 -> force_re/1
  force_im/1 -> concat/2
  force_re/1 -> concat/1

== system test_firs/fir/fir_tap_3/fir_core/tap_delay ==
  in : Inport  Port=1  LatchInput=off
  Constant : xbsIndex_r3/Constant  const=1  equ=P=C  arith_type=Boolean  n_bits=1  bin_pt=0  opselect=C  inp2=PCIN>>17  opr=+  inp1=P  carry=CIN  iostate=0  explicit_period=on  period=1  dbl_ovrd=off
  Counter : xbsIndex_r3/Counter  cnt_type=Count Limited  n_bits=6  bin_pt=0  arith_type=Unsigned  start_count=0  cnt_to=62  cnt_by_val=1  operation=Up  explicit_period=off  period=1  load_pin=off  rst=off  en=off  dbl_ovrd=off  show_param=off  use_rpm=on  gen_core=off
      settings: xl_area=[0, 0, 0, 0, 0, 0, 0]
  bram : xbsIndex_r3/Single Port RAM  depth=64  initVector=0  write_mode=Read Before Write  latency=1  init_zero=on  explicit_period=off  period=1  rst=off  init_reg=0  en=off  dbl_ovrd=off  show_param=off  distributed_mem=off  use_rpm=off  gen_core=off
      settings: xl_area=[0, 0, 0, 0, 0, 0, 0]
  out : Outport
  wires:
  Constant/1 -> bram/3
  in/1 -> bram/2
  bram/1 -> out/1
  Counter/1 -> bram/1

== system test_firs/fir/fir_tap_4/fir_coef/c_gen ==
  sync_in : Inport  Port=1  LatchInput=off
  Counter : xbsIndex_r3/Counter  cnt_type=Count Limited  n_bits=6  bin_pt=0  arith_type=Unsigned  start_count=0  cnt_to=63  cnt_by_val=1  operation=Up  explicit_period=off  period=1  load_pin=off  rst=on  en=off  dbl_ovrd=off  show_param=on  use_rpm=on  gen_core=off
      settings: xl_area=[0, 0, 0, 0, 0, 0, 0]
  addr_sel : xbsIndex_r3/Slice  mode=Upper Bit Location + Width  nbits=6  bit1=0  base1=MSB of Input  bit0=-1  base0=MSB of Input  boolean_output=off  explicit_period=off  period=1  dbl_ovrd=off
  mem : xbsIndex_r3/ROM  depth=64  initVector=[0;0;0;-0.00390625;-0.00390625;-0.00390625;-0.00390625;-0.00390625;-0.0078125;-0.0078125;-0.0078125;-0.0078125;-0.01171875;-0.01171875;-0.01171875;-0.015625;-0.015625;-0.015625;-0.01953125;-0.01953125;-0.0234375;-0.0234375;-0.0234375;-0.02734375;-0.02734375;-0.03125;-0.03125;-0.03515625;-0.0390625;-0.0390625;-0.04296875;-0.04296875;-0.046875;-0.046875;-0.05078125;-0.05078125;-0.0546875;-0.0546875;-0.05859375;-0.05859375;-0.0625;-0.0625;-0.0625;-0.0625;-0.06640625;-0.06640625;-0.06640625;-0.06640625;-0.06640625;-0.0625;-0.0625;-0.0625;-0.05859375;-0.0546875;-0.0546875;-0.05078125;-0.046875;-0.04296875;-0.0390625;-0.03125;-0.02734375;-0.01953125;-0.01171875;-0.00390625]  arith_type="Signed  (2's comp)"  n_bits=9  bin_pt=8  latency=1  init_zero=on  explicit_period=off  period=1  rst=off  init_reg=0  en=off  dbl_ovrd=off  show_param=on  distributed_mem=off  use_rpm=on  gen_core=off
      settings: AttributesFormatString=depth = %<depth>\ndist_mem = %<distributed_mem>  xl_area=[0, 0, 0, 0, 0, 0, 0]
  coef_out : Outport
  wires:
  sync_in/1 -> Counter/1
  Counter/1 -> addr_sel/1
  addr_sel/1 -> mem/1
  mem/1 -> coef_out/1

== system test_firs/fir/fir_tap_4/fir_core/c_to_ri_d ==
  c : Inport  Port=1  LatchInput=off
  force_im : xbsIndex_r3/Reinterpret  force_arith_type=on  arith_type="Signed  (2's comp)"  force_bin_pt=on  bin_pt=7  force_valid=on
  force_re : xbsIndex_r3/Reinterpret  force_arith_type=on  arith_type="Signed  (2's comp)"  force_bin_pt=on  bin_pt=7  force_valid=on
  slice_im : xbsIndex_r3/Slice  mode=Lower Bit Location + Width  nbits=8  bit1=0  base1=MSB of Input  bit0=0  base0=LSB of Input  boolean_output=off  explicit_period=off  period=1  dbl_ovrd=off
  slice_re : xbsIndex_r3/Slice  mode=Upper Bit Location + Width  nbits=8  bit1=0  base1=MSB of Input  bit0=0  base0=LSB of Input  boolean_output=off  explicit_period=off  period=1  dbl_ovrd=off
  re : Outport
  im : Outport  Port=2
  wires:
  slice_re/1 -> force_re/1
  slice_im/1 -> force_im/1
  force_re/1 -> re/1
  force_im/1 -> im/1
  c/1 -> slice_re/1, slice_im/1

== system test_firs/fir/fir_tap_4/fir_core/c_to_ri_s ==
  c : Inport  Port=1  LatchInput=off
  force_im : xbsIndex_r3/Reinterpret  force_arith_type=on  arith_type="Signed  (2's comp)"  force_bin_pt=on  bin_pt=15  force_valid=on
  force_re : xbsIndex_r3/Reinterpret  force_arith_type=on  arith_type="Signed  (2's comp)"  force_bin_pt=on  bin_pt=15  force_valid=on
  slice_im : xbsIndex_r3/Slice  mode=Lower Bit Location + Width  nbits=17  bit1=0  base1=MSB of Input  bit0=0  base0=LSB of Input  boolean_output=off  explicit_period=off  period=1  dbl_ovrd=off
  slice_re : xbsIndex_r3/Slice  mode=Upper Bit Location + Width  nbits=17  bit1=0  base1=MSB of Input  bit0=0  base0=LSB of Input  boolean_output=off  explicit_period=off  period=1  dbl_ovrd=off
  re : Outport
  im : Outport  Port=2
  wires:
  slice_re/1 -> force_re/1
  slice_im/1 -> force_im/1
  force_re/1 -> re/1
  force_im/1 -> im/1
  c/1 -> slice_re/1, slice_im/1

== system test_firs/fir/fir_tap_4/fir_core/mult_add_im ==
  a : Inport  Port=1  LatchInput=off
  b : Inport  Port=2  LatchInput=off
  c : Inport  Port=3  LatchInput=off
  add : xbsIndex_r3/AddSub  mode=Addition  precision=User Defined  arith_type="Signed  (2's comp)"  n_bits=9  bin_pt=7  quantization=Truncate  overflow=Wrap  latency=1  explicit_period=off  period=1  use_carryin=off  use_carryout=off  en=off  dbl_ovrd=off  show_param=on  use_core=on  pipeline=on  use_rpm=on  gen_core=off
      settings: xl_area=[0, 0, 0, 0, 0, 0, 0]
  delay : xbsIndex_r3/Delay  latency=3  reg_retiming=off  explicit_period=off  period=1  en=off  accept_only_valid=off  init_zero=on  dbl_ovrd=off  show_param=off
      settings: xl_area=[0, 0, 0, 0, 0, 0, 0]
  mult : xbsIndex_r3/Mult  precision=Full  arith_type="Signed  (2's comp)"  n_bits=8  bin_pt=2  quantization=Truncate  overflow=Wrap  latency=3  explicit_period=off  period=1  en=off  dbl_ovrd=off  show_param=on  mult_type=Parallel  oversample=2  use_embedded=on  pipeline=on  use_rpm=on  placement_style=Rectangular Shape  gen_core=off
      settings: xl_area=[0, 0, 0, 0, 0, 0, 0]
  out : Outport
  wires:
  add/1 -> out/1
  mult/1 -> add/1
  delay/1 -> add/2
  a/1 -> mult/1
  b/1 -> mult/2
  c/1 -> delay/1

== system test_firs/fir/fir_tap_4/fir_core/mult_add_re ==
  a : Inport  Port=1  LatchInput=off
  b : Inport  Port=2  LatchInput=off
  c : Inport  Port=3  LatchInput=off
  add : xbsIndex_r3/AddSub  mode=Addition  precision=User Defined  arith_type="Signed  (2's comp)"  n_bits=9  bin_pt=7  quantization=Truncate  overflow=Wrap  latency=1  explicit_period=off  period=1  use_carryin=off  use_carryout=off  en=off  dbl_ovrd=off  show_param=on  use_core=on  pipeline=on  use_rpm=on  gen_core=off
      settings: xl_area=[0, 0, 0, 0, 0, 0, 0]
  delay : xbsIndex_r3/Delay  latency=3  reg_retiming=off  explicit_period=off  period=1  en=off  accept_only_valid=off  init_zero=on  dbl_ovrd=off  show_param=off
      settings: xl_area=[0, 0, 0, 0, 0, 0, 0]
  mult : xbsIndex_r3/Mult  precision=Full  arith_type="Signed  (2's comp)"  n_bits=8  bin_pt=2  quantization=Truncate  overflow=Wrap  latency=3  explicit_period=off  period=1  en=off  dbl_ovrd=off  show_param=on  mult_type=Parallel  oversample=2  use_embedded=on  pipeline=on  use_rpm=on  placement_style=Rectangular Shape  gen_core=off
      settings: xl_area=[0, 0, 0, 0, 0, 0, 0]
  out : Outport
  wires:
  add/1 -> out/1
  mult/1 -> add/1
  delay/1 -> add/2
  a/1 -> mult/1
  b/1 -> mult/2
  c/1 -> delay/1

== system test_firs/fir/fir_tap_4/fir_core/ri_to_c ==
  re : Inport  Port=1  LatchInput=off
  im : Inport  Port=2  LatchInput=off
  concat : xbsIndex_r3/Concat  num_inputs=2  explicit_period=off  period=1  dbl_ovrd=off
  force_im : xbsIndex_r3/Reinterpret  force_arith_type=on  arith_type=Unsigned  force_bin_pt=on  bin_pt=0  force_valid=on
  force_re : xbsIndex_r3/Reinterpret  force_arith_type=on  arith_type=Unsigned  force_bin_pt=on  bin_pt=0  force_valid=on
  c : Outport
  wires:
  im/1 -> force_im/1
  concat/1 -> c/1
  re/1 -> force_re/1
  force_im/1 -> concat/2
  force_re/1 -> concat/1

== system test_firs/fir/fir_tap_4/fir_core/tap_delay ==
  in : Inport  Port=1  LatchInput=off
  slr : xbsIndex_r3/Delay  latency=0  reg_retiming=off  explicit_period=off  period=1  en=off  accept_only_valid=off  init_zero=on  dbl_ovrd=off  show_param=off
      settings: xl_area=[0, 0, 0, 0, 0, 0, 0]
  out : Outport
  wires:
  slr/1 -> out/1
  in/1 -> slr/1
